simulink library "conventional_airplane_aerodynamics_lib"  (R2023b)
settings: Solver=VariableStepAuto  StartTime=0.0  StopTime=10.0  RelTol=1e-3
undefined symbols (not defined in the file or in its folder): aero
libraries: simple_wing_lib x3, flight_parameters_lib x2, simpleFuselage_lib x1
settings Model: Creator=Ybeyer  LastModifiedBy=yannic
settings SolverCC: AlgebraicLoopSolver=TrustRegion
settings DataIOCC: ReturnWorkspaceOutputs=off
settings DebuggingCC: UnconnectedInputMsg=warning  UnconnectedOutputMsg=warning  UnconnectedLineMsg=warning  ArithmeticOperatorsInVariantConditions=warning
settings ModelReferenceCC: EnableRefExpFcnMdlSchedulingChecks=on
settings SFSimCC: SimUseLocalCustomCode=off  CustomCodeUndefinedFunction=UseInterfaceOnly
settings RTWCC: RTWUseLocalCustomCode=off
settings CodeAppCC: StateflowObjectComments=on

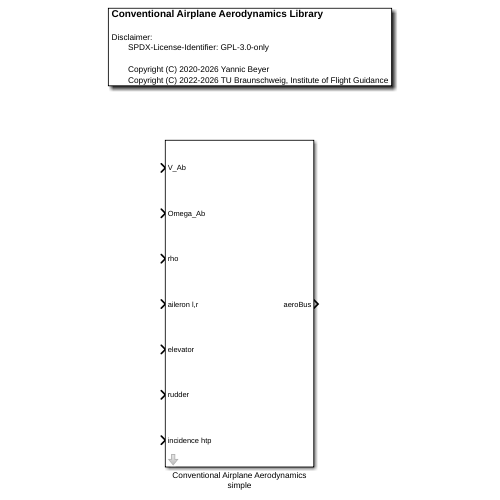
[thumbnail: Simulink's stored preview of the top-level diagram]
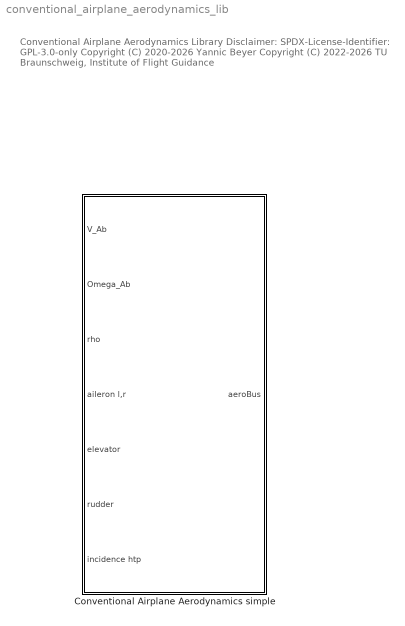
== system conventional_airplane_aerodynamics_lib ==
  note: Conventional Airplane Aerodynamics Library
      |
      | Disclaimer:
      | SPDX-License-Identifier: GPL-3.0-only
      |
      | Copyright (C) 2020-2026 Yannic Beyer
      | Copyright (C) 2022-2026 TU Braunschweig, Institute of Flight Guidance
  Conventional Airplane Aerodynamics simple : Subsystem  mask{aeroStruct=aero, xyz_cg_c=zeros(3,1)}
      mask prompts: aeroStruct "aerodynamics struct of the conventional airplane"; xyz_cg_c "center of gravity position in c frame, m"
      mask DialogControl DescGroupVar Prompt: Conventional Airplane Aerodynamics simple
      mask DialogControl DescTextVar Prompt: Contains three 2 point wing models for the main wing, the horizontal tailplane and the vertical tailplane. See conventionalAirplaneLoadParams for information about the struct.

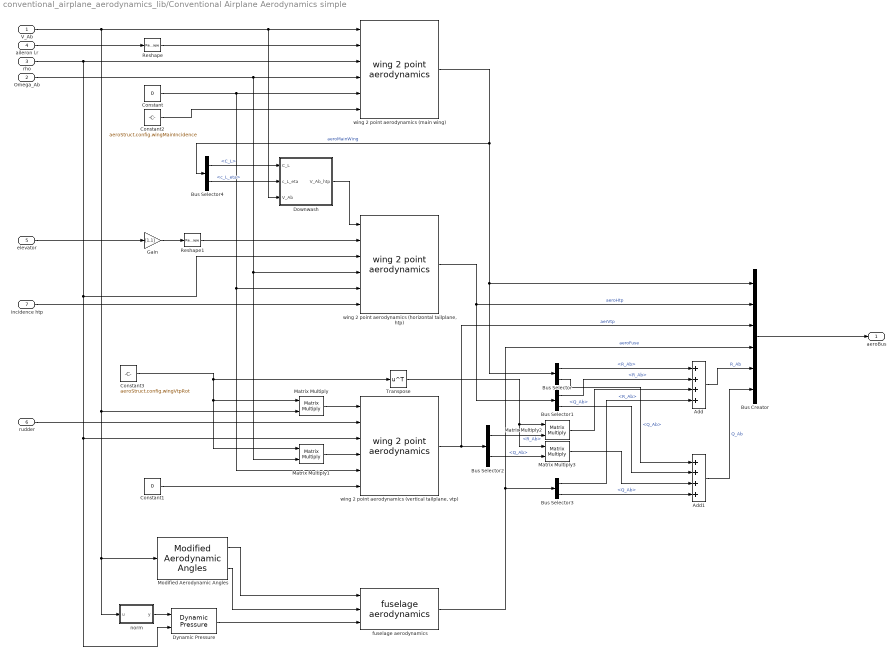
== system conventional_airplane_aerodynamics_lib/Conventional Airplane Aerodynamics simple ==
  V_Ab : Inport
  Omega_Ab : Inport  Port=2
  rho : Inport  Port=3
  aileron l,r : Inport  Port=4
  elevator : Inport  Port=5
  rudder : Inport  Port=6
  incidence htp : Inport  Port=7
  Add : Sum  Inputs=++++
  Add1 : Sum  Inputs=++++
  Bus Creator : BusCreator  Inputs=6
  Bus Selector : BusSelector  OutputSignals=dynamicsBody.R_Ab,dynamicsBody.Q_Ab
  Bus Selector1 : BusSelector  OutputSignals=dynamicsBody.R_Ab,dynamicsBody.Q_Ab
  Bus Selector2 : BusSelector  OutputSignals=dynamicsBody.R_Ab,dynamicsBody.Q_Ab
  Bus Selector3 : BusSelector  OutputSignals=R_Ab,Q_Ab
  Bus Selector4 : BusSelector  OutputSignals=dynamicsWing.C_L,dynamicsWing.c_L_eta
  Constant : Constant  Value=0
  Constant1 : Constant  Value=0
  Constant2 : Constant  Value=aeroStruct.config.wingMainIncidence
  Constant3 : Constant  Value=aeroStruct.config.wingVtpRot
  Downwash : Subsystem
  Dynamic Pressure : flight_parameters_lib/Dynamic Pressure
      settings: SourceProductName=LADAC
  Gain : Gain  Gain=[1,1]
  Matrix Multiply{,1..3} (4 alike) : Product  Multiplication=Matrix(*)
  Modified Aerodynamic Angles : flight_parameters_lib/Modified Aerodynamic Angles  SystemSampleTime=-1  VariantActivationTime=update diagram  AllowFlexibleInterface=on  Latency=0  AutoFrameSizeCalculation=off
      settings: SourceProductName=LADAC
  Reshape : Reshape  OutputDimensionality=Row vector (2-D)
  Reshape1 : Reshape  OutputDimensionality=Row vector (2-D)
  Transpose : Math  Operator=transpose  SignedPower=on
  fuselage aerodynamics : simpleFuselage_lib/fuselage aerodynamics  simple_fuselage=aeroStruct.fuse
      settings: SourceProductName=LADAC
  norm : MATLAB Function  TreatAsAtomicUnit=on
  "wing 2 point aerodynamics (horizontal tailplane, htp)" : simple_wing_lib/wing 2 point aerodynamics  wing=aeroStruct.wingHtp  xyz_wing_c=aeroStruct.config.wingHtpPos  xyz_cg_c=xyz_cg_c
      settings: SourceProductName=LADAC
  wing 2 point aerodynamics (main wing) : simple_wing_lib/wing 2 point aerodynamics  wing=aeroStruct.wingMain  xyz_wing_c=aeroStruct.config.wingMainPos  xyz_cg_c=xyz_cg_c
      settings: SourceProductName=LADAC
  "wing 2 point aerodynamics (vertical tailplane, vtp)" : simple_wing_lib/wing 2 point aerodynamics  wing=aeroStruct.wingVtp  xyz_wing_c=aeroStruct.config.wingVtpRot*aeroStruct.config.wingVtpPos  xyz_cg_c=aeroStruct.config.wingVtpRot*xyz_cg_c
      settings: SourceProductName=LADAC
  aeroBus : Outport  VectorParamsAs1DForOutWhenUnconnected=off
  wires:
  V_Ab/1 -> Matrix Multiply/2, norm/1(u), Modified Aerodynamic Angles/1, Downwash/3(V_Ab), wing 2 point aerodynamics (main wing)/1
  aileron l,r/1 -> Reshape/1
  rho/1 -> wing 2 point aerodynamics (main wing)/3, "wing 2 point aerodynamics (horizontal tailplane, htp)"/3, Dynamic Pressure/2, "wing 2 point aerodynamics (vertical tailplane, vtp)"/3
  Dynamic Pressure/1 -> fuselage aerodynamics/3
  Constant/1 -> wing 2 point aerodynamics (main wing)/5, "wing 2 point aerodynamics (vertical tailplane, vtp)"/5, "wing 2 point aerodynamics (horizontal tailplane, htp)"/5
  Constant2/1 -> wing 2 point aerodynamics (main wing)/6
  incidence htp/1 -> "wing 2 point aerodynamics (horizontal tailplane, htp)"/6
  Constant1/1 -> "wing 2 point aerodynamics (vertical tailplane, vtp)"/6
  Modified Aerodynamic Angles/1 -> fuselage aerodynamics/1
  Modified Aerodynamic Angles/2 -> fuselage aerodynamics/2
  norm/1(y) -> Dynamic Pressure/1
  elevator/1 -> Gain/1
  Gain/1 -> Reshape1/1
  rudder/1 -> "wing 2 point aerodynamics (vertical tailplane, vtp)"/2
  wing 2 point aerodynamics (main wing)/1 -> Bus Selector/1, Bus Creator/1, Bus Selector4/1  "aeroMainWing"
  "wing 2 point aerodynamics (horizontal tailplane, htp)"/1 -> Bus Creator/2, Bus Selector1/1  "aeroHtp"
  "wing 2 point aerodynamics (vertical tailplane, vtp)"/1 -> Bus Creator/3, Bus Selector2/1  "aerVtp"
  Bus Creator/1 -> aeroBus/1
  fuselage aerodynamics/1 -> Bus Creator/4, Bus Selector3/1  "aeroFuse"
  Reshape/1 -> wing 2 point aerodynamics (main wing)/2
  Reshape1/1 -> "wing 2 point aerodynamics (horizontal tailplane, htp)"/2
  Matrix Multiply/1 -> "wing 2 point aerodynamics (vertical tailplane, vtp)"/1
  Constant3/1 -> Matrix Multiply1/1, Matrix Multiply/1, Transpose/1
  Matrix Multiply1/1 -> "wing 2 point aerodynamics (vertical tailplane, vtp)"/4
  Omega_Ab/1 -> wing 2 point aerodynamics (main wing)/4, Matrix Multiply1/2, "wing 2 point aerodynamics (horizontal tailplane, htp)"/4
  Bus Selector/1 -> Add/1  "<R_Ab>"
  Bus Selector1/1 -> Add/2  "<R_Ab>"
  Matrix Multiply2/1 -> Add/3
  Bus Selector3/1 -> Add/4  "<R_Ab>"
  Bus Selector3/2 -> Add1/4  "<Q_Ab>"
  Matrix Multiply3/1 -> Add1/3
  Bus Selector1/2 -> Add1/2  "<Q_Ab>"
  Bus Selector/2 -> Add1/1  "<Q_Ab>"
  Add/1 -> Bus Creator/5  "R_Ab"
  Add1/1 -> Bus Creator/6  "Q_Ab"
  Bus Selector2/1 -> Matrix Multiply2/2  "<R_Ab>"
  Bus Selector2/2 -> Matrix Multiply3/2  "<Q_Ab>"
  Transpose/1 -> Matrix Multiply3/1, Matrix Multiply2/1
  Bus Selector4/1 -> Downwash/1(C_L)  "<C_L>"
  Bus Selector4/2 -> Downwash/2(c_L_eta)  "<c_L_eta>"
  Downwash/1(V_Ab_htp) -> "wing 2 point aerodynamics (horizontal tailplane, htp)"/1

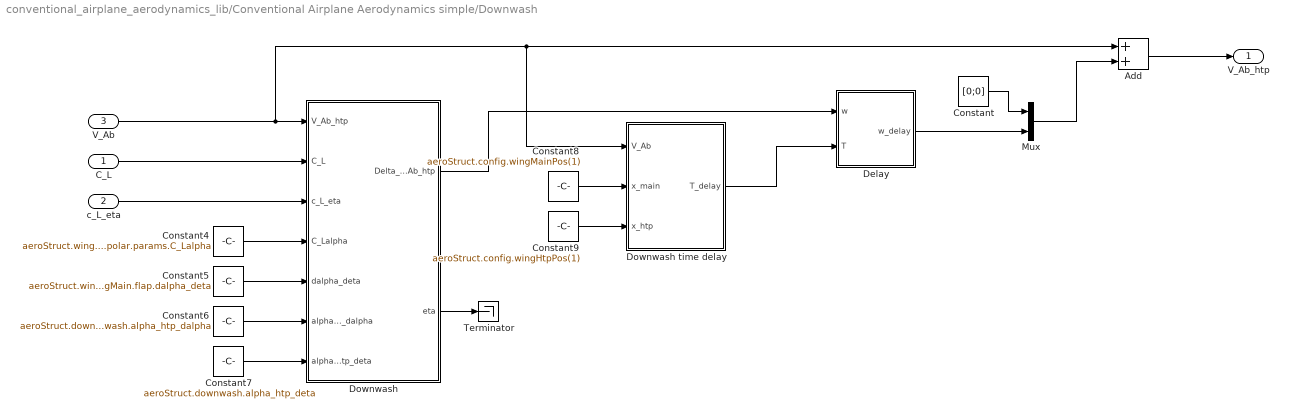
== system conventional_airplane_aerodynamics_lib/Conventional Airplane Aerodynamics simple/Downwash ==
  C_L : Inport
  c_L_eta : Inport  Port=2
  V_Ab : Inport  Port=3
  Add : Sum
  Constant : Constant  Value=[0;0]  VectorParams1D=off
  Constant4 : Constant  Value=aeroStruct.wingMain.polar.params.C_Lalpha
  Constant5 : Constant  Value=aeroStruct.wingMain.flap.dalpha_deta
  Constant6 : Constant  Value=aeroStruct.downwash.alpha_htp_dalpha
  Constant7 : Constant  Value=aeroStruct.downwash.alpha_htp_deta
  Constant8 : Constant  Value=aeroStruct.config.wingMainPos(1)
  Constant9 : Constant  Value=aeroStruct.config.wingHtpPos(1)
  Delay : Subsystem
  Downwash : MATLAB Function  TreatAsAtomicUnit=on
  Downwash time delay : MATLAB Function  TreatAsAtomicUnit=on
  Mux : Mux  Inputs=2
  Terminator : Terminator
  V_Ab_htp : Outport  VectorParamsAs1DForOutWhenUnconnected=off
  wires:
  Constant7/1 -> Downwash/7(alpha_htp_deta)
  Constant5/1 -> Downwash/5(dalpha_deta)
  Constant6/1 -> Downwash/6(alpha_htp_dalpha)
  Constant4/1 -> Downwash/4(C_Lalpha)
  C_L/1 -> Downwash/2(C_L)
  Constant8/1 -> Downwash time delay/2(x_main)
  Constant9/1 -> Downwash time delay/3(x_htp)
  c_L_eta/1 -> Downwash/3(c_L_eta)
  V_Ab/1 -> Downwash time delay/1(V_Ab), Add/1, Downwash/1(V_Ab_htp)
  Downwash time delay/1(T_delay) -> Delay/2(T)
  Downwash/1(Delta_w_Ab_htp) -> Delay/1(w)
  Add/1 -> V_Ab_htp/1
  Delay/1(w_delay) -> Mux/2
  Downwash/2(eta) -> Terminator/1
  Constant/1 -> Mux/1
  Mux/1 -> Add/2

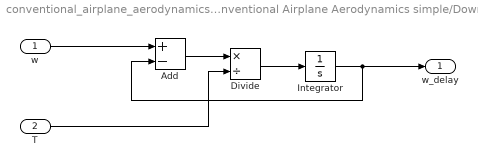
== system conventional_airplane_aerodynamics_lib/Conventional Airplane Aerodynamics simple/Downwash/Delay ==
  w : Inport
  T : Inport  Port=2
  Add : Sum  Inputs=+-
  Divide : Product  Inputs=*/
  Integrator : Integrator
  w_delay : Outport
  wires:
  w/1 -> Add/1
  Add/1 -> Divide/1
  Divide/1 -> Integrator/1
  Integrator/1 -> Add/2, w_delay/1
  T/1 -> Divide/2

== matlab function conventional_airplane_aerodynamics_lib/Conventional Airplane Aerodynamics simple/norm ==
  data: u input; y output
function y = fcn(u)
y = norm(u,2);

== matlab function conventional_airplane_aerodynamics_lib/Conventional Airplane Aerodynamics simple/Downwash/Downwash ==
  data: V_Ab_htp input; Delta_w_Ab_htp output; C_L input; c_L_eta input; C_Lalpha input; dalpha_deta input; alpha_htp_dalpha input; alpha_htp_deta input; eta output
function [Delta_w_Ab_htp,eta] = fcn(V_Ab_htp,C_L, c_L_eta, C_Lalpha, dalpha_deta, alpha_htp_dalpha, alpha_htp_deta)
C_L_alpha = mean(C_L) - sum(c_L_eta);
% downwash due to main wing lift
alpha = C_L_alpha / C_Lalpha;
alpha_htp = alpha_htp_dalpha(:)' * alpha;
eta = c_L_eta ./ (C_Lalpha * dalpha_deta(:)');
% add downwash due to main wing flap deflections
alpha_htp = alpha_htp + sum(alpha_htp_deta(:)' .* eta);
% reduce downwash in case of high aerodynamic angles
u_Ab_rel = divideFinite( V_Ab_htp(1), norm(V_Ab_htp) );
cos_arg = 3 * pi/2*(1-u_Ab_rel);
cos_arg(abs(cos_arg)>pi/2) = pi/2;    
alpha_htp = alpha_htp * cos(cos_arg);
% vertical velocity at HTP
Delta_w_Ab_htp = alpha_htp*V_Ab_htp(1);
end

== matlab function conventional_airplane_aerodynamics_lib/Conventional Airplane Aerodynamics simple/Downwash/Downwash time delay ==
  data: V_Ab input; x_main input; T_delay output; x_htp input
function T_delay = fcn(V_Ab, x_main, x_htp)
T_delay = divideFinite( x_main - x_htp, V_Ab(1) );
% avoid singularity
T_delay(T_delay<0.001) = 0.001;
end
